simulink model "HandMove"  (R2021a)
settings: Solver=ode1  StartTime=0.0  StopTime=20  FixedStep=.002  RelTol=1e-3  EnableMultiTasking=on
libraries: QB_pacer_lib x1, qbmove_library_2017a x1, qbmove_library x1, simulink x1
settings Model: Creator=laurentio  LastModifiedBy=sohei
settings SolverCC: AlgebraicLoopSolver=TrustRegion
settings DataIOCC: LimitDataPoints=on  SaveFormat=Array  ReturnWorkspaceOutputs=off
settings OptimizationCC: LifeSpan=inf
settings DebuggingCC: UnderspecifiedInitializationDetection=Classic  MergeDetectMultiDrivingBlocksExec=none  SolverPrmCheckMsg=warning  AllowSymbolicDim=off  StateNameClashWarn=warning  SFUnexpectedBacktrackingDiag=warning  SFNoUnconditionalDefaultTransitionDiag=warning  SFExecutionAtInitializationDiag=none  SFMachineParentedDataDiag=warning  ArithmeticOperatorsInVariantConditions=warning
settings HardwareCC: ProdBitPerPointer=32  ProdBitPerSizeT=32  ProdBitPerPtrDiffT=32  ProdLargestAtomicFloat=None  ProdIntDivRoundTo=Undefined  ProdEndianess=Unspecified  ProdWordSize=32  ProdHWDeviceType=32-bit Generic
settings ModelReferenceCC: PropagateSignalLabelsOutOfModel=off
settings SFSimCC: SimUseLocalCustomCode=off  CustomCodeUndefinedFunction=UseInterfaceOnly
settings RTWCC: RTWUseLocalCustomCode=off
settings CodeAppCC: StateflowObjectComments=on
settings GRTTargetCC: TargetLangStandard=C89/C90 (ANSI)
settings ConfigComp: CovMetricSettings=dw  CovSaveCumulativeToWorkspaceVar=on  CovSaveSingleToWorkspaceVar=on  CovExternalEMLEnable=off  CovSFcnEnable=off

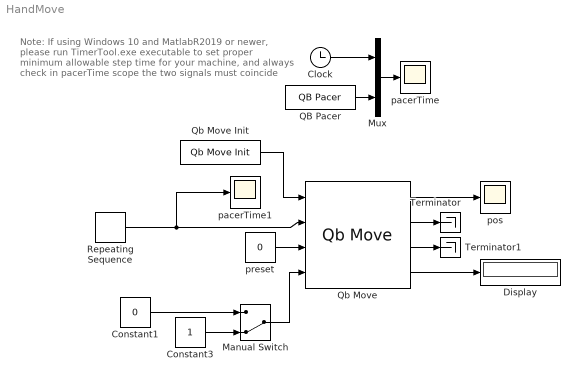
== system HandMove ==
  note: Note: If using Windows 10 and MatlabR2019 or newer,
      | please run TimerTool.exe executable to set
      | proper minimum allowable step time for your machine,
      | and always check in pacerTime scope the two signals
      | must coincide
  Clock : Clock
  Constant1 : Constant  Value=0
  Constant3 : Constant
  Display : Display
  Manual Switch : ManualSwitch  CurrentSetting=0
  Mux : Mux  Inputs=2
  QB Pacer : QB_pacer_lib/QB Pacer  simTimePerRealTime=1
      settings: SourceProductName=QB Pacer
  Qb Move : qbmove_library_2017a/Qb Move  ID=1  ACTIVE_COMM_DIRECTIONS=Both  CONTROL_MODE=Prime Movers Positions  DAISY_CHAINING=off  MAX_ANG=0  SW_LIMIT=inf  OFFSET=0  ACTIVATE=off  WDT=0.0  UNIT=TICK
      settings: SourceProductName=Qb Move Library
  Qb Move Init : qbmove_library/Qb Move Init  NUMBER_OF_COM='COM6'  BAUD_RATE_COM=2000000
      settings: SourceProductName=Qb Move Library
  Repeating Sequence : simulink/Sources/Repeating Sequence  rep_seq_t="[0  10  20]"  rep_seq_y="[0 10000  0]"
  Terminator : Terminator
  Terminator1 : Terminator
  pacerTime : Scope
  pacerTime1 : Scope
  pos : Scope
  preset : Constant  Value=0
  wires:
  QB Pacer/1 -> Mux/2
  Clock/1 -> Mux/1
  Qb Move Init/1 -> Qb Move/1
  Constant1/1 -> Manual Switch/1
  Repeating Sequence/1 -> pacerTime1/1, Qb Move/2
  Constant3/1 -> Manual Switch/2
  preset/1 -> Qb Move/3
  Qb Move/4 -> Display/1
  Mux/1 -> pacerTime/1
  Manual Switch/1 -> Qb Move/4
  Qb Move/1 -> pos/1
  Qb Move/2 -> Terminator/1
  Qb Move/3 -> Terminator1/1
